simulink model "Aero_UltraStick25e"  (R2016b)
settings: Solver=VariableStepAuto  StartTime=0.0  StopTime=10.0  RelTol=1e-3
undefined symbols (not defined in the file or in its folder): AC
libraries: simulink x1
settings Model: Creator=UAVLAB  LastModifiedBy=rega0051

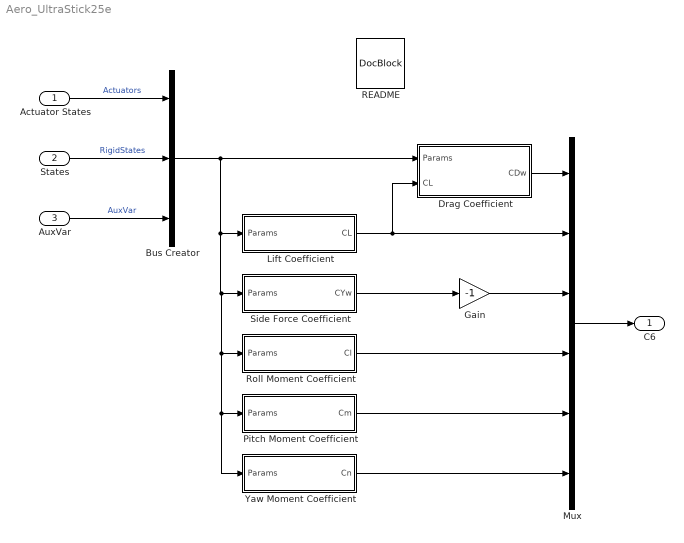
== system Aero_UltraStick25e ==
  Actuator States : Inport  OutDataTypeStr=Bus: Actuators
  States : Inport  Port=2  OutDataTypeStr=Bus: RigidStates
  AuxVar : Inport  Port=3  OutDataTypeStr=Bus: AuxVar
  Bus Creator : BusCreator  Inputs=3
  Drag Coefficient : Subsystem
  Gain : Gain  Gain=-1
  Lift Coefficient : Subsystem
  Mux : Mux  Inputs=6
  Pitch Moment Coefficient : Subsystem
  README : simulink/Model-Wide Utilities/DocBlock  DocumentType=Text
      content=|
      | Ultrastick Aerodynamic Model
      |
      | This block models the Ultrastick aerodynamics using a linear derivatives.
      | The force coefficients are in the wind axes, but the moment coefficients
      | are in body axes, so the six coefficients are CL, CDw, CYw, Cl, Cm, Cn.
      | See Klein, Morelli, Aircraft System Identification, pg 41. Thus in the
      | Aero lib, the force and moment transformation block must be set as though
      | outgoing moment coefficients are in wind axes so no transformation is
      | applied.
      |
      | The derivatives are stored in the aircraft configuration data structure
      | (AC). They are loaded into AC.Aero when 'Ulstrastick' is selected with
      | UAV_config.m.  The derivatives themselves are stored in
      | Ultrastick_config.m. An example is the derivatives for CL:
      |
      | >>  AC.Aero.CL
      |
      | ans =
      |
      |         zero: 0.1086
      |        alpha: 4.5800
      |        dflap: 0.7400
      |        delev: 0.0983
      |     alphadot: 1.9724
      |            q: 6.1639
      |         minD: 0.2300
      |
      | The majority of the derivatives have been indentified from flight test
      | data. The drag model was derived from first principles.
  Roll Moment Coefficient : Subsystem
  Side Force Coefficient : Subsystem
  Yaw Moment Coefficient : Subsystem
  C6 : Outport
  wires:
  Mux/1 -> C6/1
  Yaw Moment Coefficient/1(Cn) -> Mux/6
  Pitch Moment Coefficient/1(Cm) -> Mux/5
  Roll Moment Coefficient/1(Cl) -> Mux/4
  Drag Coefficient/1(CDw) -> Mux/1
  States/1 -> Bus Creator/2  "RigidStates"
  Lift Coefficient/1(CL) -> Drag Coefficient/2(CL), Mux/2
  AuxVar/1 -> Bus Creator/3  "AuxVar"
  Actuator States/1 -> Bus Creator/1  "Actuators"
  Side Force Coefficient/1(CYw) -> Gain/1
  Bus Creator/1 -> Lift Coefficient/1(Params), Yaw Moment Coefficient/1(Params), Pitch Moment Coefficient/1(Params), Roll Moment Coefficient/1(Params), Side Force Coefficient/1(Params), Drag Coefficient/1(Params)
  Gain/1 -> Mux/3

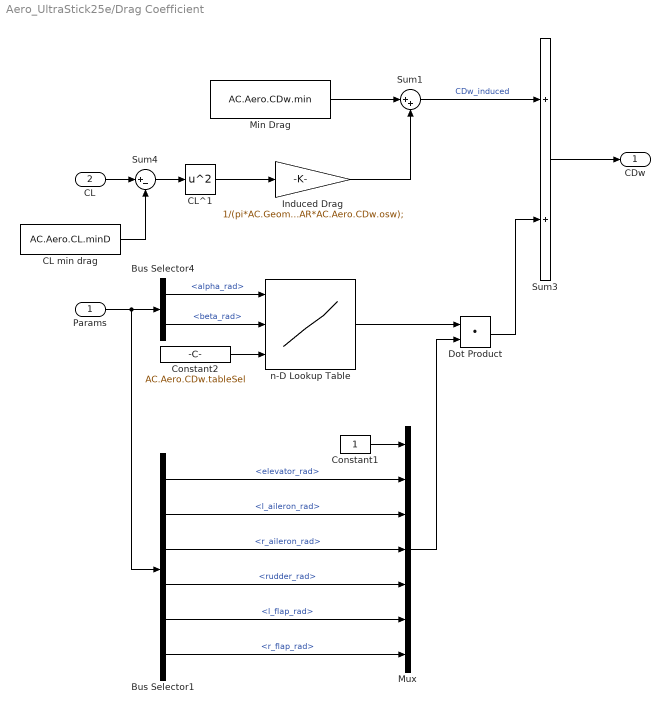
== system Aero_UltraStick25e/Drag Coefficient ==
  Params : Inport
  CL : Inport  Port=2
  Bus Selector1 : BusSelector  OutputSignals=Actuators.CtrlSurf.elevator_rad,Actuators.CtrlSurf.l_aileron_rad,Actuators.CtrlSurf.r_aileron_rad,Actuators.CtrlSurf.rudder_rad,Actuators.CtrlSurf.l_flap_rad,Actuators.CtrlSurf.r_flap_rad
  Bus Selector4 : BusSelector  OutputSignals=AuxVar.WindAxesParams.alpha_rad,AuxVar.WindAxesParams.beta_rad
  CL min drag : Constant  Value=AC.Aero.CL.minD
  CL^1 : Math  Operator=square  SaturateOnIntegerOverflow=on
  Constant1 : Constant
  Constant2 : Constant  Value=AC.Aero.CDw.tableSel
      settings: AttributesFormatString=%<Value>
  Dot Product : DotProduct  InputSameDT=on  OutDataTypeStr=Inherit: Inherit via internal rule
  Induced Drag : Gain  Gain=1/(pi*AC.Geometry.AR*AC.Aero.CDw.osw);  SaturateOnIntegerOverflow=on  OutDataTypeStr=Inherit: Same as input  ParamDataTypeStr=Inherit: Same as input
      settings: AttributesFormatString=%<Gain>
  Min Drag : Constant  Value=AC.Aero.CDw.min
  Mux : Mux  Inputs=length(AC.Aero.CDw.tableSel)
  Sum1 : Sum  Inputs=|++  SaturateOnIntegerOverflow=on  InputSameDT=on  OutDataTypeStr=Inherit: Same as first input
  Sum3 : Sum  SaturateOnIntegerOverflow=on  InputSameDT=on  OutDataTypeStr=Inherit: Same as first input
  Sum4 : Sum  Inputs=|+-  SaturateOnIntegerOverflow=on  InputSameDT=on  OutDataTypeStr=Inherit: Same as first input
  n-D Lookup Table : Lookup_n-D  NumberOfTableDimensions=3  BreakpointsForDimension1=AC.Aero.CDw.breakPts{1}  BreakpointsForDimension2=AC.Aero.CDw.breakPts{2}  BreakpointsForDimension3=AC.Aero.CDw.tableSel  Table=AC.Aero.CDw.table  InternalRulePriority=Speed  RndMeth=Simplest  InputSameDT=on
      settings: AttributesFormatString=%<Table>
  CDw : Outport
  wires:
  Min Drag/1 -> Sum1/1
  Sum3/1 -> CDw/1
  Induced Drag/1 -> Sum1/2
  CL^1/1 -> Induced Drag/1
  Sum4/1 -> CL^1/1
  CL min drag/1 -> Sum4/2
  CL/1 -> Sum4/1
  Mux/1 -> Dot Product/2
  Bus Selector4/2 -> n-D Lookup Table/2  "<beta_rad>"
  Constant2/1 -> n-D Lookup Table/3
  Dot Product/1 -> Sum3/2
  Params/1 -> Bus Selector1/1, Bus Selector4/1
  Bus Selector4/1 -> n-D Lookup Table/1  "<alpha_rad>"
  Constant1/1 -> Mux/1
  n-D Lookup Table/1 -> Dot Product/1
  Bus Selector1/1 -> Mux/2  "<elevator_rad>"
  Bus Selector1/2 -> Mux/3  "<l_aileron_rad>"
  Bus Selector1/3 -> Mux/4  "<r_aileron_rad>"
  Bus Selector1/4 -> Mux/5  "<rudder_rad>"
  Bus Selector1/5 -> Mux/6  "<l_flap_rad>"
  Bus Selector1/6 -> Mux/7  "<r_flap_rad>"
  Sum1/1 -> Sum3/1  "CDw_induced"

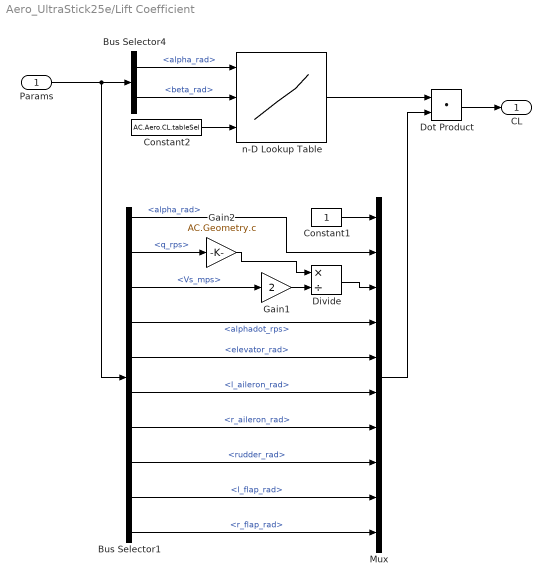
== system Aero_UltraStick25e/Lift Coefficient ==
  Params : Inport
  Bus Selector1 : BusSelector  OutputSignals=AuxVar.WindAxesParams.alpha_rad,RigidStates.AngVel.q_rps,AuxVar.WindAxesParams.Vs_mps,AuxVar.AlphaBetaDot.alphadot_rps,Actuators.CtrlSurf.elevator_rad,Actuators.CtrlSurf.l_aileron_rad,Actuators.CtrlSurf.r_aileron_rad,Actuators.CtrlSurf.rudder_rad,Actuators.CtrlSurf.l_flap_rad,Actuators.CtrlSurf.r_flap_rad
  Bus Selector4 : BusSelector  OutputSignals=AuxVar.WindAxesParams.alpha_rad,AuxVar.WindAxesParams.beta_rad
  Constant1 : Constant
  Constant2 : Constant  Value=AC.Aero.CL.tableSel
      settings: AttributesFormatString=%<Value>
  Divide : Product  Inputs=*/
  Dot Product : DotProduct  InputSameDT=on  OutDataTypeStr=Inherit: Inherit via internal rule
  Gain1 : Gain  Gain=2  SaturateOnIntegerOverflow=on  OutDataTypeStr=Inherit: Same as input  ParamDataTypeStr=Inherit: Same as input
  Gain2 : Gain  Gain=AC.Geometry.c  SaturateOnIntegerOverflow=on  OutDataTypeStr=Inherit: Same as input  ParamDataTypeStr=Inherit: Same as input
      settings: AttributesFormatString=%<Gain>
  Mux : Mux  Inputs=length(AC.Aero.CL.tableSel)
  n-D Lookup Table : Lookup_n-D  NumberOfTableDimensions=3  BreakpointsForDimension1=AC.Aero.CL.breakPts{1}  BreakpointsForDimension2=AC.Aero.CL.breakPts{2}  BreakpointsForDimension3=AC.Aero.CL.tableSel  Table=AC.Aero.CL.table  InternalRulePriority=Speed  RndMeth=Simplest  InputSameDT=on
      settings: AttributesFormatString=%<Table>
  CL : Outport
  wires:
  Dot Product/1 -> CL/1
  Bus Selector4/1 -> n-D Lookup Table/1  "<alpha_rad>"
  Bus Selector4/2 -> n-D Lookup Table/2  "<beta_rad>"
  Params/1 -> Bus Selector4/1, Bus Selector1/1
  Gain2/1 -> Divide/1
  Constant2/1 -> n-D Lookup Table/3
  n-D Lookup Table/1 -> Dot Product/1
  Mux/1 -> Dot Product/2
  Constant1/1 -> Mux/1
  Gain1/1 -> Divide/2
  Divide/1 -> Mux/3
  Bus Selector1/1 -> Mux/2  "<alpha_rad>"
  Bus Selector1/2 -> Gain2/1  "<q_rps>"
  Bus Selector1/3 -> Gain1/1  "<Vs_mps>"
  Bus Selector1/5 -> Mux/5  "<elevator_rad>"
  Bus Selector1/4 -> Mux/4  "<alphadot_rps>"
  Bus Selector1/6 -> Mux/6  "<l_aileron_rad>"
  Bus Selector1/7 -> Mux/7  "<r_aileron_rad>"
  Bus Selector1/8 -> Mux/8  "<rudder_rad>"
  Bus Selector1/9 -> Mux/9  "<l_flap_rad>"
  Bus Selector1/10 -> Mux/10  "<r_flap_rad>"

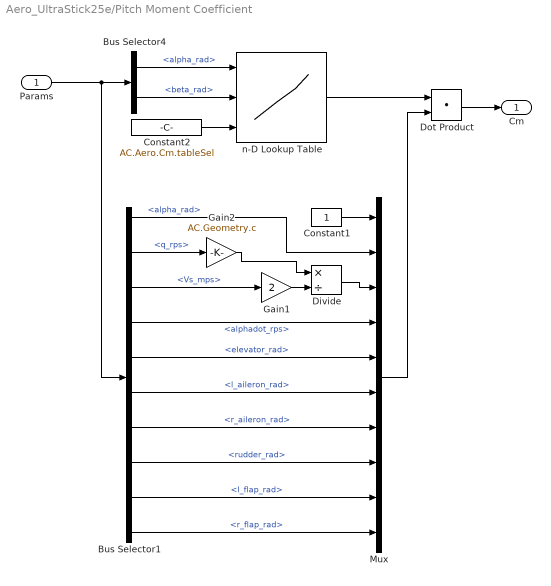
== system Aero_UltraStick25e/Pitch Moment Coefficient ==
  Params : Inport
  Bus Selector1 : BusSelector  OutputSignals=AuxVar.WindAxesParams.alpha_rad,RigidStates.AngVel.q_rps,AuxVar.WindAxesParams.Vs_mps,AuxVar.AlphaBetaDot.alphadot_rps,Actuators.CtrlSurf.elevator_rad,Actuators.CtrlSurf.l_aileron_rad,Actuators.CtrlSurf.r_aileron_rad,Actuators.CtrlSurf.rudder_rad,Actuators.CtrlSurf.l_flap_rad,Actuators.CtrlSurf.r_flap_rad
  Bus Selector4 : BusSelector  OutputSignals=AuxVar.WindAxesParams.alpha_rad,AuxVar.WindAxesParams.beta_rad
  Constant1 : Constant
  Constant2 : Constant  Value=AC.Aero.Cm.tableSel
      settings: AttributesFormatString=%<Value>
  Divide : Product  Inputs=*/
  Dot Product : DotProduct  InputSameDT=on  OutDataTypeStr=Inherit: Inherit via internal rule
  Gain1 : Gain  Gain=2  SaturateOnIntegerOverflow=on  OutDataTypeStr=Inherit: Same as input  ParamDataTypeStr=Inherit: Same as input
  Gain2 : Gain  Gain=AC.Geometry.c  SaturateOnIntegerOverflow=on  OutDataTypeStr=Inherit: Same as input  ParamDataTypeStr=Inherit: Same as input
      settings: AttributesFormatString=%<Gain>
  Mux : Mux  Inputs=length(AC.Aero.Cm.tableSel)
  n-D Lookup Table : Lookup_n-D  NumberOfTableDimensions=3  BreakpointsForDimension1=AC.Aero.Cm.breakPts{1}  BreakpointsForDimension2=AC.Aero.Cm.breakPts{2}  BreakpointsForDimension3=AC.Aero.Cm.tableSel  Table=AC.Aero.Cm.table  InternalRulePriority=Speed  RndMeth=Simplest  InputSameDT=on
      settings: AttributesFormatString=%<Table>
  Cm : Outport
  wires:
  Bus Selector1/10 -> Mux/10  "<r_flap_rad>"
  Bus Selector1/9 -> Mux/9  "<l_flap_rad>"
  Bus Selector1/8 -> Mux/8  "<rudder_rad>"
  Bus Selector1/7 -> Mux/7  "<r_aileron_rad>"
  Bus Selector1/6 -> Mux/6  "<l_aileron_rad>"
  Bus Selector1/5 -> Mux/5  "<elevator_rad>"
  Bus Selector1/3 -> Gain1/1  "<Vs_mps>"
  Bus Selector1/2 -> Gain2/1  "<q_rps>"
  Bus Selector1/1 -> Mux/2  "<alpha_rad>"
  Divide/1 -> Mux/3
  Gain1/1 -> Divide/2
  Constant1/1 -> Mux/1
  Mux/1 -> Dot Product/2
  n-D Lookup Table/1 -> Dot Product/1
  Constant2/1 -> n-D Lookup Table/3
  Gain2/1 -> Divide/1
  Params/1 -> Bus Selector1/1, Bus Selector4/1
  Bus Selector4/2 -> n-D Lookup Table/2  "<beta_rad>"
  Bus Selector4/1 -> n-D Lookup Table/1  "<alpha_rad>"
  Dot Product/1 -> Cm/1
  Bus Selector1/4 -> Mux/4  "<alphadot_rps>"

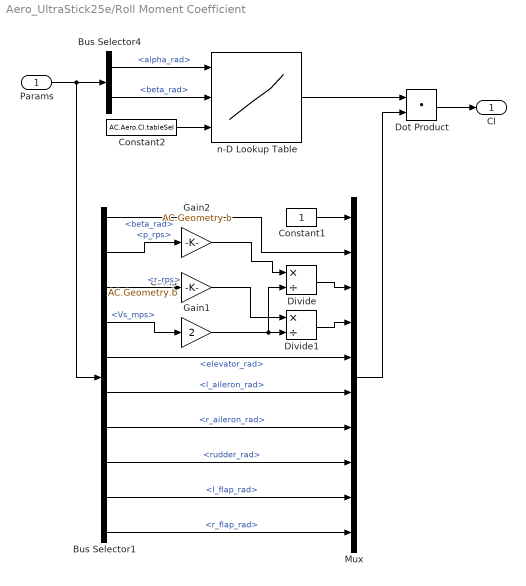
== system Aero_UltraStick25e/Roll Moment Coefficient ==
  Params : Inport
  Bus Selector1 : BusSelector  OutputSignals=AuxVar.WindAxesParams.beta_rad,RigidStates.AngVel.p_rps,RigidStates.AngVel.r_rps,AuxVar.WindAxesParams.Vs_mps,Actuators.CtrlSurf.elevator_rad,Actuators.CtrlSurf.l_aileron_rad,Actuators.CtrlSurf.r_aileron_rad,Actuators.CtrlSurf.rudder_rad,Actuators.CtrlSurf.l_flap_rad,Actuators.CtrlSurf.r_flap_rad
  Bus Selector4 : BusSelector  OutputSignals=AuxVar.WindAxesParams.alpha_rad,AuxVar.WindAxesParams.beta_rad
  Constant1 : Constant
  Constant2 : Constant  Value=AC.Aero.Cl.tableSel
      settings: AttributesFormatString=%<Value>
  Divide : Product  Inputs=*/
  Divide1 : Product  Inputs=*/
  Dot Product : DotProduct  InputSameDT=on  OutDataTypeStr=Inherit: Inherit via internal rule
  Gain1 : Gain  Gain=2  SaturateOnIntegerOverflow=on  OutDataTypeStr=Inherit: Same as input  ParamDataTypeStr=Inherit: Same as input
  Gain2 : Gain  Gain=AC.Geometry.b  SaturateOnIntegerOverflow=on  OutDataTypeStr=Inherit: Same as input  ParamDataTypeStr=Inherit: Same as input
      settings: AttributesFormatString=%<Gain>
  Gain3 : Gain  Gain=AC.Geometry.b  SaturateOnIntegerOverflow=on  OutDataTypeStr=Inherit: Same as input  ParamDataTypeStr=Inherit: Same as input
      settings: AttributesFormatString=%<Gain>
  Mux : Mux  Inputs=length(AC.Aero.Cl.tableSel)
  n-D Lookup Table : Lookup_n-D  NumberOfTableDimensions=3  BreakpointsForDimension1=AC.Aero.Cl.breakPts{1}  BreakpointsForDimension2=AC.Aero.Cl.breakPts{2}  BreakpointsForDimension3=AC.Aero.Cl.tableSel  Table=AC.Aero.Cl.table  InternalRulePriority=Speed  RndMeth=Simplest  InputSameDT=on
      settings: AttributesFormatString=%<Table>
  Cl : Outport
  wires:
  Mux/1 -> Dot Product/2
  Bus Selector1/4 -> Gain1/1  "<Vs_mps>"
  Gain1/1 -> Divide/2, Divide1/2
  Bus Selector1/5 -> Mux/5  "<elevator_rad>"
  Bus Selector4/2 -> n-D Lookup Table/2  "<beta_rad>"
  Constant2/1 -> n-D Lookup Table/3
  Bus Selector1/2 -> Gain2/1  "<p_rps>"
  Bus Selector1/9 -> Mux/9  "<l_flap_rad>"
  Bus Selector1/10 -> Mux/10  "<r_flap_rad>"
  Dot Product/1 -> Cl/1
  Params/1 -> Bus Selector4/1, Bus Selector1/1
  Gain2/1 -> Divide/1
  Bus Selector1/8 -> Mux/8  "<rudder_rad>"
  Bus Selector4/1 -> n-D Lookup Table/1  "<alpha_rad>"
  Constant1/1 -> Mux/1
  Bus Selector1/1 -> Mux/2  "<beta_rad>"
  Divide/1 -> Mux/3
  Bus Selector1/6 -> Mux/6  "<l_aileron_rad>"
  n-D Lookup Table/1 -> Dot Product/1
  Bus Selector1/7 -> Mux/7  "<r_aileron_rad>"
  Bus Selector1/3 -> Gain3/1  "<r_rps>"
  Gain3/1 -> Divide1/1
  Divide1/1 -> Mux/4

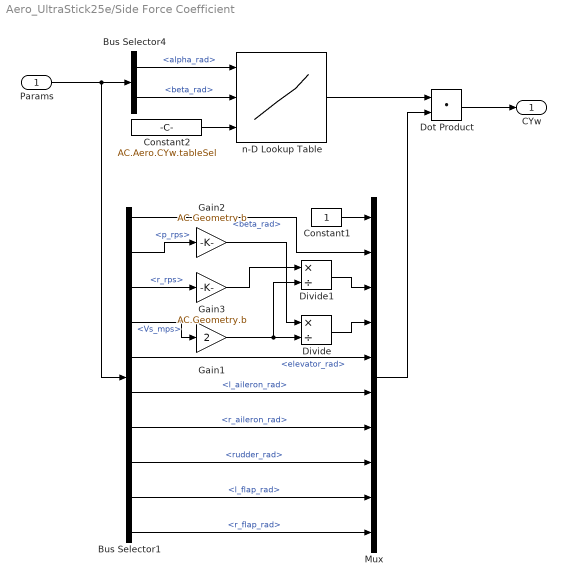
== system Aero_UltraStick25e/Side Force Coefficient ==
  Params : Inport
  Bus Selector1 : BusSelector  OutputSignals=AuxVar.WindAxesParams.beta_rad,RigidStates.AngVel.p_rps,RigidStates.AngVel.r_rps,AuxVar.WindAxesParams.Vs_mps,Actuators.CtrlSurf.elevator_rad,Actuators.CtrlSurf.l_aileron_rad,Actuators.CtrlSurf.r_aileron_rad,Actuators.CtrlSurf.rudder_rad,Actuators.CtrlSurf.l_flap_rad,Actuators.CtrlSurf.r_flap_rad
  Bus Selector4 : BusSelector  OutputSignals=AuxVar.WindAxesParams.alpha_rad,AuxVar.WindAxesParams.beta_rad
  Constant1 : Constant
  Constant2 : Constant  Value=AC.Aero.CYw.tableSel
      settings: AttributesFormatString=%<Value>
  Divide : Product  Inputs=*/
  Divide1 : Product  Inputs=*/
  Dot Product : DotProduct  InputSameDT=on  OutDataTypeStr=Inherit: Inherit via internal rule
  Gain1 : Gain  Gain=2  SaturateOnIntegerOverflow=on  OutDataTypeStr=Inherit: Same as input  ParamDataTypeStr=Inherit: Same as input
  Gain2 : Gain  Gain=AC.Geometry.b  SaturateOnIntegerOverflow=on  OutDataTypeStr=Inherit: Same as input  ParamDataTypeStr=Inherit: Same as input
      settings: AttributesFormatString=%<Gain>
  Gain3 : Gain  Gain=AC.Geometry.b  SaturateOnIntegerOverflow=on  OutDataTypeStr=Inherit: Same as input  ParamDataTypeStr=Inherit: Same as input
      settings: AttributesFormatString=%<Gain>
  Mux : Mux  Inputs=length(AC.Aero.CYw.tableSel)
  n-D Lookup Table : Lookup_n-D  NumberOfTableDimensions=3  BreakpointsForDimension1=AC.Aero.CYw.breakPts{1}  BreakpointsForDimension2=AC.Aero.CYw.breakPts{2}  BreakpointsForDimension3=AC.Aero.CYw.tableSel  Table=AC.Aero.CYw.table  InternalRulePriority=Speed  RndMeth=Simplest  InputSameDT=on
      settings: AttributesFormatString=%<Table>
  CYw : Outport
  wires:
  Dot Product/1 -> CYw/1
  Mux/1 -> Dot Product/2
  Bus Selector1/4 -> Gain1/1  "<Vs_mps>"
  Gain1/1 -> Divide1/2, Divide/2
  Bus Selector1/5 -> Mux/5  "<elevator_rad>"
  Bus Selector4/2 -> n-D Lookup Table/2  "<beta_rad>"
  Constant2/1 -> n-D Lookup Table/3
  Bus Selector1/2 -> Gain2/1  "<p_rps>"
  Bus Selector1/9 -> Mux/9  "<l_flap_rad>"
  Bus Selector1/10 -> Mux/10  "<r_flap_rad>"
  Gain2/1 -> Divide/1
  Bus Selector1/8 -> Mux/8  "<rudder_rad>"
  Bus Selector4/1 -> n-D Lookup Table/1  "<alpha_rad>"
  Constant1/1 -> Mux/1
  Bus Selector1/6 -> Mux/6  "<l_aileron_rad>"
  n-D Lookup Table/1 -> Dot Product/1
  Bus Selector1/7 -> Mux/7  "<r_aileron_rad>"
  Params/1 -> Bus Selector4/1, Bus Selector1/1
  Divide/1 -> Mux/4
  Divide1/1 -> Mux/3
  Bus Selector1/3 -> Gain3/1  "<r_rps>"
  Gain3/1 -> Divide1/1
  Bus Selector1/1 -> Mux/2  "<beta_rad>"

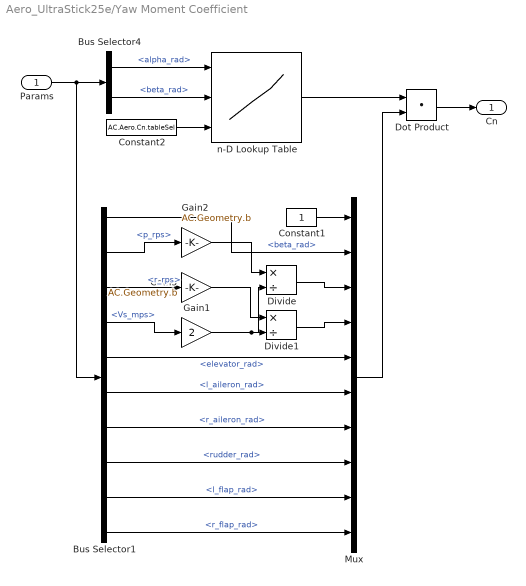
== system Aero_UltraStick25e/Yaw Moment Coefficient ==
  Params : Inport
  Bus Selector1 : BusSelector  OutputSignals=AuxVar.WindAxesParams.beta_rad,RigidStates.AngVel.p_rps,RigidStates.AngVel.r_rps,AuxVar.WindAxesParams.Vs_mps,Actuators.CtrlSurf.elevator_rad,Actuators.CtrlSurf.l_aileron_rad,Actuators.CtrlSurf.r_aileron_rad,Actuators.CtrlSurf.rudder_rad,Actuators.CtrlSurf.l_flap_rad,Actuators.CtrlSurf.r_flap_rad
  Bus Selector4 : BusSelector  OutputSignals=AuxVar.WindAxesParams.alpha_rad,AuxVar.WindAxesParams.beta_rad
  Constant1 : Constant
  Constant2 : Constant  Value=AC.Aero.Cn.tableSel
      settings: AttributesFormatString=%<Value>
  Divide : Product  Inputs=*/
  Divide1 : Product  Inputs=*/
  Dot Product : DotProduct  InputSameDT=on  OutDataTypeStr=Inherit: Inherit via internal rule
  Gain1 : Gain  Gain=2  SaturateOnIntegerOverflow=on  OutDataTypeStr=Inherit: Same as input  ParamDataTypeStr=Inherit: Same as input
  Gain2 : Gain  Gain=AC.Geometry.b  SaturateOnIntegerOverflow=on  OutDataTypeStr=Inherit: Same as input  ParamDataTypeStr=Inherit: Same as input
      settings: AttributesFormatString=%<Gain>
  Gain3 : Gain  Gain=AC.Geometry.b  SaturateOnIntegerOverflow=on  OutDataTypeStr=Inherit: Same as input  ParamDataTypeStr=Inherit: Same as input
      settings: AttributesFormatString=%<Gain>
  Mux : Mux  Inputs=length(AC.Aero.Cn.tableSel)
  n-D Lookup Table : Lookup_n-D  NumberOfTableDimensions=3  BreakpointsForDimension1=AC.Aero.Cn.breakPts{1}  BreakpointsForDimension2=AC.Aero.Cn.breakPts{2}  BreakpointsForDimension3=AC.Aero.Cn.tableSel  Table=AC.Aero.Cn.table  InternalRulePriority=Speed  RndMeth=Simplest  InputSameDT=on
      settings: AttributesFormatString=%<Table>
  Cn : Outport
  wires:
  Mux/1 -> Dot Product/2
  Bus Selector1/4 -> Gain1/1  "<Vs_mps>"
  Gain1/1 -> Divide/2, Divide1/2
  Bus Selector4/2 -> n-D Lookup Table/2  "<beta_rad>"
  Constant2/1 -> n-D Lookup Table/3
  Bus Selector1/2 -> Gain2/1  "<p_rps>"
  Dot Product/1 -> Cn/1
  Params/1 -> Bus Selector4/1, Bus Selector1/1
  Gain2/1 -> Divide/1
  Bus Selector4/1 -> n-D Lookup Table/1  "<alpha_rad>"
  Constant1/1 -> Mux/1
  n-D Lookup Table/1 -> Dot Product/1
  Bus Selector1/3 -> Gain3/1  "<r_rps>"
  Gain3/1 -> Divide1/1
  Bus Selector1/1 -> Mux/2  "<beta_rad>"
  Divide/1 -> Mux/3
  Divide1/1 -> Mux/4
  Bus Selector1/6 -> Mux/6  "<l_aileron_rad>"
  Bus Selector1/7 -> Mux/7  "<r_aileron_rad>"
  Bus Selector1/8 -> Mux/8  "<rudder_rad>"
  Bus Selector1/9 -> Mux/9  "<l_flap_rad>"
  Bus Selector1/10 -> Mux/10  "<r_flap_rad>"
  Bus Selector1/5 -> Mux/5  "<elevator_rad>"
